simulink model "dspwwv_synchronization_template"  (Simulink 8.3)
settings: Solver=FixedStepDiscrete  StartTime=0.0  StopTime=10.0  RelTol=1e-3
libraries: dspbuff3 x1, dspmisc x1
settings Model: Creator=The MathWorks Inc.
settings OptimizationCC: ExpressionDepthLimit=2147483647  InitFltsAndDblsToZero=on
settings DebuggingCC: FcnCallInpInsideContextMsg=UseLocalSettings  StrictBusMsg=Warning

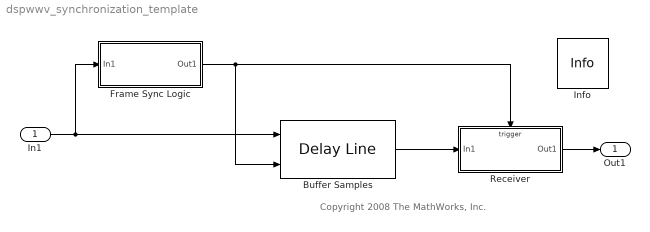
== system dspwwv_synchronization_template ==
  note: Copyright 2008 The MathWorks, Inc.
  In1 : Inport  SampleTime=1
  Buffer Samples : dspbuff3/Delay Line  siz=64  ic=0  directfeed=off  enable_output=on  hold_output=off  TreatMby1Signals=One channel
  Frame Sync Logic : Subsystem
  Info : dspmisc/Info  SystemSampleTime=-1
  Receiver : Subsystem  TreatAsAtomicUnit=on
  Out1 : Outport
  wires:
  In1/1 -> Buffer Samples/1, Frame Sync Logic/1(In1)
  Buffer Samples/1 -> Receiver/1(In1)
  Receiver/1(Out1) -> Out1/1
  Frame Sync Logic/1(Out1) -> Receiver/Trigger, Buffer Samples/2

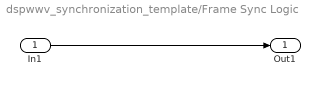
== system dspwwv_synchronization_template/Frame Sync Logic ==
  In1 : Inport
  Out1 : Outport
  wires:
  In1/1 -> Out1/1

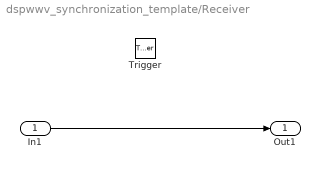
== system dspwwv_synchronization_template/Receiver ==
  In1 : Inport
  Trigger : TriggerPort
  Out1 : Outport
  wires:
  In1/1 -> Out1/1
